simulink model "imu_6dof"  (R2020b)
settings: Solver=VariableStepAuto  StartTime=0.0  StopTime=10.0  RelTol=1e-3
model mask{sample_rate=100, a_sf_cc=[1, 0, 0; 0, 1, 0; 0, 0, 1], a_bias=[0 0 0], a_noise=[0 0 0], a_sath=[inf inf inf], a_satl=[-inf -inf -inf], g_sf_cc=[1, 0, 0; 0, 1, 0; 0, 0, 1], g_sen=[0 0 0], g_bias=[0 0 0], g_noise=[0 0 0], g_sath=[inf inf inf], g_satl=[-inf -inf -inf]}
  mask prompts: sample_rate "Sample Rate [Hz]:"; a_sf_cc "Scale factors and cross coupling:"; a_bias "Bias [m/s/s]:"; a_noise "Noise [m/s/s]:"; a_sath "Upper limits [m/s/s]:"; a_satl "Lower limits [m/s/s]:"; g_sf_cc "Scale factors and cross coupling:"; g_sen "G-sensitivity [rad/s per m/s/s]:"; g_bias "Bias [rad/s]:"; g_noise "Noise [rad/s]:"; g_sath "Upper limits [rad/s]:"; g_satl "Lower limits [rad/s]:"
model workspace (MAT data in the model file):
  a_bias = Simulink.Parameter
  a_bias.Value = [0 0 0]
  a_bias.DataType = 'auto'
  a_bias.Dimensions = [1 3]
  a_noise = Simulink.Parameter
  a_noise.Value = [0 0 0]
  a_noise.DataType = 'auto'
  a_noise.Dimensions = [1 3]
  a_sath = Simulink.Parameter
  a_sath.Value = [Inf Inf Inf]
  a_sath.DataType = 'auto'
  a_sath.Dimensions = [1 3]
  a_satl = Simulink.Parameter
  a_satl.Value = [-Inf -Inf -Inf]
  a_satl.DataType = 'auto'
  a_satl.Dimensions = [1 3]
  a_sf_cc = Simulink.Parameter
  a_sf_cc.Value = [1  0  0; 0  1  0; 0  0  1]
  a_sf_cc.DataType = 'auto'
  a_sf_cc.Dimensions = [3 3]
  g_bias = Simulink.Parameter
  g_bias.Value = [0 0 0]
  g_bias.DataType = 'auto'
  g_bias.Dimensions = [1 3]
  g_noise = Simulink.Parameter
  g_noise.Value = [0 0 0]
  g_noise.DataType = 'auto'
  g_noise.Dimensions = [1 3]
  g_sath = Simulink.Parameter
  g_sath.Value = [Inf Inf Inf]
  g_sath.DataType = 'auto'
  g_sath.Dimensions = [1 3]
  g_satl = Simulink.Parameter
  g_satl.Value = [0 0 0]
  g_satl.DataType = 'auto'
  g_satl.Dimensions = [1 3]
  g_sen = Simulink.Parameter
  g_sen.Value = [0 0 0]
  g_sen.DataType = 'auto'
  g_sen.Dimensions = [1 3]
  g_sf_cc = Simulink.Parameter
  g_sf_cc.Value = [1  0  0; 0  1  0; 0  0  1]
  g_sf_cc.DataType = 'auto'
  g_sf_cc.Dimensions = [3 3]
  sample_rate = Simulink.Parameter
  sample_rate.Value = 100
  sample_rate.DataType = 'auto'
  sample_rate.Dimensions = [1 1]
settings Model: ParameterArgumentNames=a_bias,a_noise,a_sath,a_satl,a_sf_cc,g_bias,g_noise,g_sath,g_satl,g_sen,g_sf_cc,sample_rate  OrderedModelArguments=off  Creator=brian  LastModifiedBy=brian

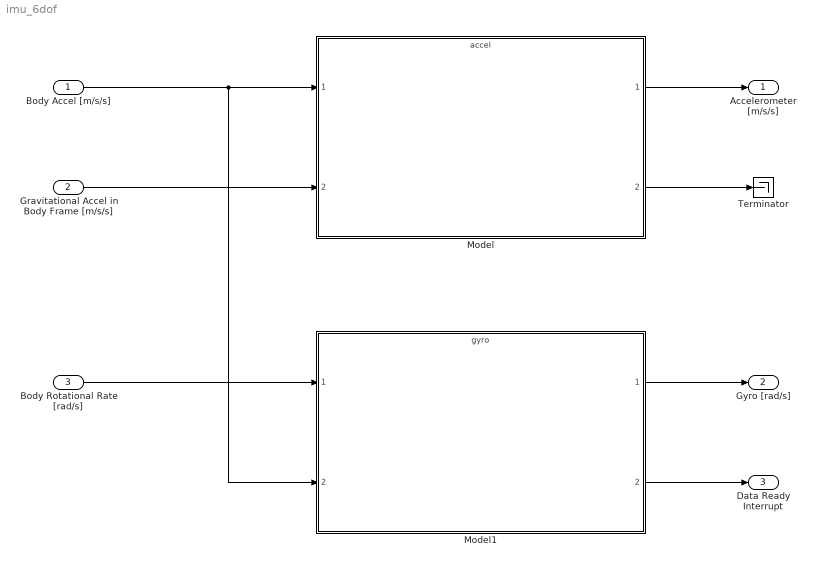
== system imu_6dof ==
  Body Accel [m/s/s] : Inport
  Gravitational Accel in Body Frame [m/s/s] : Inport  Port=2
  Body Rotational Rate [rad/s] : Inport  Port=3
  Model : ModelReference  ModelNameDialog=accel.slx  UsingDefaultArgumentValue=0,0,0,0,0,0  SimulationMode=Normal  ModelReferenceVersion=1.28  a_sf_cc=a_sf_cc  a_bias=a_bias  a_noise=a_noise  a_sath=a_sath  a_satl=a_satl  sample_rate=sample_rate  SimulationMode=Normal
  Model1 : ModelReference  ModelNameDialog=gyro.slx  UsingDefaultArgumentValue=0,0,0,0,0,0,0  SimulationMode=Normal  ModelReferenceVersion=1.23  g_sf_cc=g_sf_cc  g_sen=g_sen  g_bias=g_bias  g_noise=g_noise  g_sath=g_sath  g_satl=g_satl  sample_rate=sample_rate  SimulationMode=Normal
  Terminator : Terminator
  Accelerometer [m/s/s] : Outport
  Gyro [rad/s] : Outport  Port=2
  Data Ready Interrupt : Outport  Port=3
  wires:
  Model/2 -> Terminator/1
  Model/1 -> Accelerometer [m/s/s]/1
  Model1/1 -> Gyro [rad/s]/1
  Model1/2 -> Data Ready Interrupt/1
  Body Rotational Rate [rad/s]/1 -> Model1/1
  Gravitational Accel in Body Frame [m/s/s]/1 -> Model/2
  Body Accel [m/s/s]/1 -> Model1/2, Model/1
